simulink model "P2005_230215_CumulativeCostEMEffectsVector"  (R2022b)
settings: Solver=VariableStepAuto  StartTime=0.0  StopTime=10  RelTol=1e-7
values from neighbouring files (symbols this model uses):
  p0 = 0.2 * (ii - 1)    [P2005_230215_CumulativeCostEMEffectOfp0Vector.m]
settings Model: Creator=turib  LastModifiedBy=turib
settings HardwareCC: ProdHWDeviceType=AMD->x86-64 (Windows64)

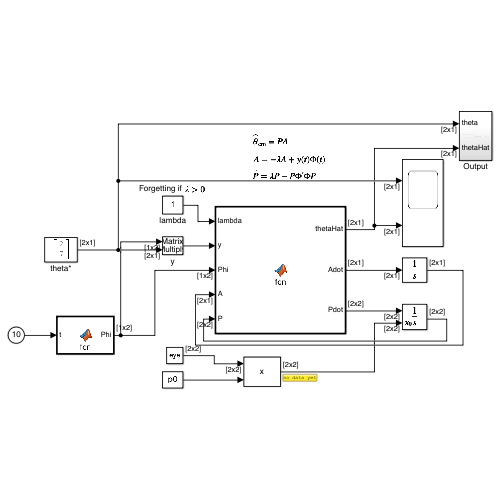
[thumbnail: Simulink's stored preview of the top-level diagram]
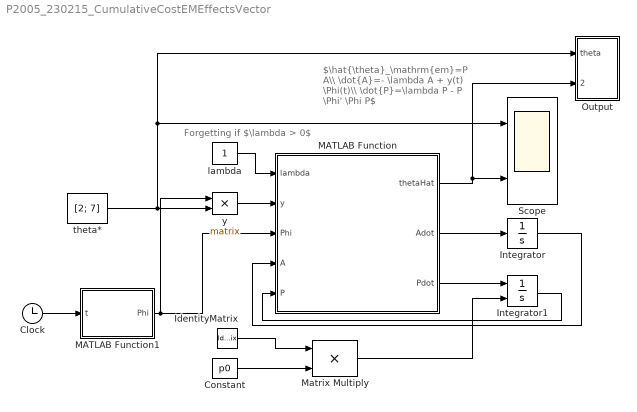
== system P2005_230215_CumulativeCostEMEffectsVector ==
  note: Forgetting if $\lambda > 0$
  note: $\hat{\theta}_\mathrm{em}=P A\\ \dot{A}=- \lambda A + y(t) \Phi(t)\\ \dot{P}=\lambda P - P \Phi' \Phi P$
  Clock : Clock
  Constant : Constant  Value=p0
  IdentityMatrix : IdentityMatrix  OutputDimensions=2
  Integrator : Integrator  InitialCondition=[0;0]
  Integrator1 : Integrator  InitialConditionSource=external  InitialCondition=1
  MATLAB Function : MATLAB Function  TreatAsAtomicUnit=on
  MATLAB Function1 : MATLAB Function  TreatAsAtomicUnit=on
  Matrix Multiply : Product
  Output : Subsystem
  Scope : Scope  NumInputPorts=2
  lambda : Constant
  theta* : Constant  Value=[2; 7]  VectorParams1D=off
  y : Product  Multiplication=Matrix(*)  OutDataTypeStr=double
  wires:
  y/1 -> MATLAB Function/2(y)
  theta*/1 -> Output/1(theta), Scope/1, y/2
  Clock/1 -> MATLAB Function1/1(t)
  MATLAB Function1/1(Phi) -> MATLAB Function/3(Phi), y/1
  lambda/1 -> MATLAB Function/1(lambda)
  IdentityMatrix/1 -> Matrix Multiply/1
  Constant/1 -> Matrix Multiply/2
  MATLAB Function/1(thetaHat) -> Output/2(thetaHat), Scope/2
  MATLAB Function/2(Adot) -> Integrator/1
  MATLAB Function/3(Pdot) -> Integrator1/1
  Matrix Multiply/1 -> Integrator1/2
  Integrator1/1 -> MATLAB Function/5(P)
  Integrator/1 -> MATLAB Function/4(A)

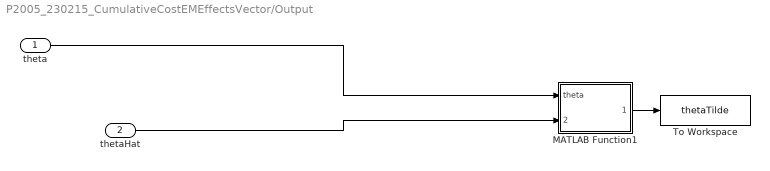
== system P2005_230215_CumulativeCostEMEffectsVector/Output ==
  theta : Inport
  thetaHat : Inport  Port=2
  MATLAB Function1 : MATLAB Function  TreatAsAtomicUnit=on
  To Workspace : ToWorkspace  VariableName=thetaTilde  SampleTime=-1
  wires:
  MATLAB Function1/1(thetaTilde) -> To Workspace/1
  thetaHat/1 -> MATLAB Function1/2(thetaHat)
  theta/1 -> MATLAB Function1/1(theta)

== matlab function P2005_230215_CumulativeCostEMEffectsVector/Output/MATLAB Function1 ==
  data: theta input; thetaTilde output; thetaHat input
function thetaTilde = error(theta, thetaHat)

thetaTilde = norm(thetaHat - theta);

end

== matlab function P2005_230215_CumulativeCostEMEffectsVector/MATLAB Function ==
  data: thetaHat output; lambda input; Adot output; y input; Phi input; A input; P input; Pdot output
function [thetaHat, Adot, Pdot] = fcn(lambda, y, Phi, ...
    A, P)

thetaHat = P * A;
Adot = - lambda * A + Phi' * y;
Pdot = lambda * P - P * Phi' * Phi * P;
% B = inv(P);
% Jder = -2 * (A - B * thetaHat);

end

== matlab function P2005_230215_CumulativeCostEMEffectsVector/MATLAB Function1 ==
  data: t input; Phi output
function Phi = fcn(t)

Phi = [sin(t), cos(t)];

end
